simulink model "RefModel_Task"  (R2015b)
settings: configuration reference "CenterOutReachConfigSet" (kept outside this file)
undefined symbols (not defined in the file or in its folder): SimulinkParameter_TunableConditionRepeats, SimulinkParameter_TunableConditions, SimulinkParameter_TunableDataLoggerInfo, SimulinkParameter_TunableNextTrialId, SimulinkParameter_TunableParam, SimulinkParameter_TunableTaskControl
libraries: libBusSerialize x7, libUtilities x1, dspsrcs4 x1
(part 1 of 3)
settings Model: SimulationMode=external  Creator=djoshea  LastModifiedBy=shenoylab
settings ConfigSetRef: SourceLocation=Base Workspace

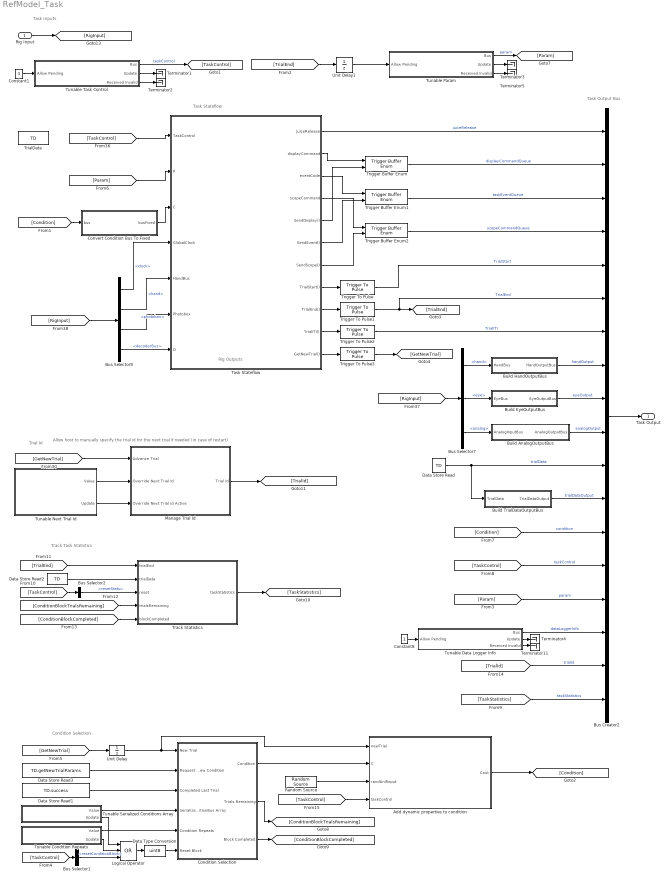
== system RefModel_Task ==
  note: Task Stateflow
  note: Rig Outputs
  note: Task Inputs
  note: Condition Selection
  note: Trial Id
  note: Allow host to manually specify the trial id for the next trial if needed (in case of restart)
  note: Track Task Statistics
  note: Task Output Bus
  Rig Input : Inport  OutDataTypeStr=Bus: RigInputBus  PortDimensions=1  SampleTime=[0.001,0]  Interpolate=off  BusOutputAsStruct=on
  Add dynamic properties to condition : MATLAB Function  TreatAsAtomicUnit=on
  Build AnalogOutputBus : Subsystem
  Build EyeOutputBus : Subsystem
  Build HandOutputBus : Subsystem
  Build TrialDataOutputBus : Subsystem
  Bus Creator2 : BusCreator  Inputs=18
  Bus Selector1 : BusSelector  OutputSignals=resetConditionBlock
  Bus Selector2 : BusSelector  OutputSignals=resetStats
  Bus Selector7 : BusSelector  OutputSignals=hand,eye,analog
  Bus Selector9 : BusSelector  OutputSignals=clock,hand,analog.photobox,decoderBus
  Condition Selection : Subsystem
  Constant1 : Constant  OutDataTypeStr=uint8
  Constant8 : Constant  OutDataTypeStr=uint8
  Convert Condition Bus To Fixed : MATLAB Function  AncestorBlock=libBusSerialize/MATLAB Function1  TreatAsAtomicUnit=on  mask(Drop Variable Length Signals From Bus){busType=Bus: ConditionBus, busFixedType=Bus: ConditionFixedBus}
      mask prompts: busType "Bus Type (Input):"; busFixedType "Bus Type (Output):"
      mask help:
      | This block takes as input a bus with some variable length signals, drops all variable length signals from the bus and outputs a bus with the specified type (second drop-down). This is accomplished by calling the appropriate model packaged code function for this bus.
      |
      | See BusSerialize.createBusBaseWorkspaceWithFixedSizeSignalsOnly and BusSerialize.writeDropVariableLengthSignalsFromBusModelPackagedCode.
      mask init:
      | BusSerialize.maskDropVariableLengthSignalsFromBusBlockUpdate(gcb)
  Data Store Read : DataStoreRead  DataStoreName=TD
  Data Store Read1 : DataStoreRead  DataStoreName=TD  DataStoreElements=TD.success
  Data Store Read2 : DataStoreRead  DataStoreName=TD
  Data Store Read3 : DataStoreRead  DataStoreName=TD  DataStoreElements=TD.getNewTrialParams
  Data Type Conversion : DataTypeConversion  OutDataTypeStr=uint8
  Logical Operator : Logic  Operator=OR  Inputs=3  AllPortsSameDT=off  OutDataTypeStr=boolean
  Manage Trial Id : Subsystem
  Random Source : dspsrcs4/Random Source  SrcType=Uniform  NormMethod=Ziggurat  CltLength=12  MinVal=0  MaxVal=1  MeanVal=0  VarVal=1  RepMode=Not repeatable  rawSeed=1  IsInherit=off  SampMode=Discrete  SampTime=0.001  SampFrame=1  DataType=Double  OutComplex=Real  OutputFrames=on
  Task Stateflow : Stateflow chart  TreatAsAtomicUnit=on
  Terminator{1..5,11} (6 alike) : Terminator
  Track Statistics : MATLAB Function  TreatAsAtomicUnit=on
  TrialData : DataStoreMemory  DataStoreName=TD  ReadBeforeWriteMsg=warning  WriteAfterWriteMsg=warning  WriteAfterReadMsg=warning  OutDataTypeStr=Bus: TrialDataBus
  Trigger Buffer Enum : libBusSerialize/Trigger Buffer Enum  bufferType=Enum: DisplayCommand
  Trigger Buffer Enum1 : libBusSerialize/Trigger Buffer Enum  bufferType=Enum: TaskEvent
  Trigger Buffer Enum2 : libBusSerialize/Trigger Buffer Enum  bufferType=Enum: ScopeCommand
  Trigger To Pulse{,1..3} (4 alike) : libBusSerialize/Trigger To Pulse
  Tunable Condition Repeats : Subsystem  AncestorBlock=libBusSerialize/Tunable Parameter  mask(BusSerialize Tunable Parameter Block){paramName='TunableConditionRepeats'}
      mask prompts: paramName "Parameter Name"
      mask help: This block provides the value of a tunable Simulink.Parameter into the model. Since tunable parameters with xPC target can only be doubles, the functions BusSerialize.createTunableParameter and BusSerialize.setTunableParameter automatically handle typecasting and update counter insertion, and this block handles update detection, typecasting, and reshaping back to the original form. Currently, variable size parameters are not supported.
      mask init:
      | BusSerialize.maskTunableParameterBlockUpdate(gcb);
      mask Display:
      | port_label('output', 1, paramName)
      | port_label('output', 2, 'Update');
  Tunable Data Logger Info : Subsystem  AncestorBlock=libBusSerialize/Serialized Bus Tunable Parameter  mask(BusSerialize Tunable Parameter Block){paramName='TunableDataLoggerInfo'}
      mask prompts: paramName "Parameter Name"
      mask help: This block provides the value of a tunable Simulink.Parameter into the model. Since tunable parameters with xPC target can only be doubles, the functions BusSerialize.createTunableParameter and BusSerialize.setTunableParameter automatically handle typecasting and update counter insertion, and this block handles update detection, typecasting, and reshaping back to the original form. Currently, variable size parameters are not supported.
      mask init:
      | BusSerialize.maskSerializedBusTunableParameterBlockUpdate(gcb);
      mask Display:
      | port_label('output', 1, paramName);
      | port_label('output', 2, 'Update');
      | port_label('output', 3, 'Received Invalid');
      | port_label('input', 1, 'Allow Pending');
  Tunable Next Trial Id : Subsystem  AncestorBlock=libBusSerialize/Tunable Parameter  mask(BusSerialize Tunable Parameter Block){paramName='TunableNextTrialId'}
      mask prompts: paramName "Parameter Name"
      mask help: This block provides the value of a tunable Simulink.Parameter into the model. Since tunable parameters with xPC target can only be doubles, the functions BusSerialize.createTunableParameter and BusSerialize.setTunableParameter automatically handle typecasting and update counter insertion, and this block handles update detection, typecasting, and reshaping back to the original form. Currently, variable size parameters are not supported.
      mask init:
      | BusSerialize.maskTunableParameterBlockUpdate(gcb);
      mask Display:
      | port_label('output', 1, paramName)
      | port_label('output', 2, 'Update');
  Tunable Param : Subsystem  AncestorBlock=libBusSerialize/Serialized Bus Tunable Parameter  mask(BusSerialize Tunable Parameter Block){paramName='TunableParam'}
      mask prompts: paramName "Parameter Name"
      mask help: This block provides the value of a tunable Simulink.Parameter into the model. Since tunable parameters with xPC target can only be doubles, the functions BusSerialize.createTunableParameter and BusSerialize.setTunableParameter automatically handle typecasting and update counter insertion, and this block handles update detection, typecasting, and reshaping back to the original form. Currently, variable size parameters are not supported.
      mask init:
      | BusSerialize.maskSerializedBusTunableParameterBlockUpdate(gcb);
      mask Display:
      | port_label('output', 1, paramName);
      | port_label('output', 2, 'Update');
      | port_label('output', 3, 'Received Invalid');
      | port_label('input', 1, 'Allow Pending');
  Tunable Serialized Conditions Array : Subsystem  AncestorBlock=libBusSerialize/Tunable Serialized Conditions Array  mask(BusSerialize Tunable Parameter Variable Length Bus Array Block){paramName='TunableConditions'}
      mask prompts: paramName "Parameter Name"
      mask help:
      | This block provides the value of a tunable Simulink.Parameter into the model. Since tunable parameters with xPC target can only be doubles, the functions BusSerialize.createTunableParameter and BusSerialize.setTunableParameter automatically handle typecasting and update counter insertion, and this block handles update detection, typecasting, and reshaping back to the original form. Currently, variable size parameters are not supported.
      |
      | This block specifically extracts a serialized variable length bus array, which can then be passed into the variable length bus array element extractor block.
      mask init:
      | BusSerialize.maskTunableParameterVariableLengthBusArrayBlockUpdate(gcb);
      mask Display:
      | port_label('output', 1, paramName)
      | port_label('output', 2, 'Update');
  Tunable Task Control : Subsystem  AncestorBlock=libBusSerialize/Serialized Bus Tunable Parameter  mask(BusSerialize Tunable Parameter Block){paramName='TunableTaskControl'}
      mask prompts: paramName "Parameter Name"
      mask help: This block provides the value of a tunable Simulink.Parameter into the model. Since tunable parameters with xPC target can only be doubles, the functions BusSerialize.createTunableParameter and BusSerialize.setTunableParameter automatically handle typecasting and update counter insertion, and this block handles update detection, typecasting, and reshaping back to the original form. Currently, variable size parameters are not supported.
      mask init:
      | BusSerialize.maskSerializedBusTunableParameterBlockUpdate(gcb);
      mask Display:
      | port_label('output', 1, paramName);
      | port_label('output', 2, 'Update');
      | port_label('output', 3, 'Received Invalid');
      | port_label('input', 1, 'Allow Pending');
  Unit Delay : UnitDelay  SampleTime=-1
  Unit Delay1 : UnitDelay  SampleTime=-1
  Task Output : Outport  OutDataTypeStr=Bus: TaskOutputBus  PortDimensions=1  SampleTime=[0.001,0]  BusOutputAsStruct=on
  wires:
  Task Stateflow/5(SendDisplay()) -> Trigger Buffer Enum/2
  Task Stateflow/9(TrialEnd()) -> Trigger To Pulse1/1
  Rig Input/1 -> [RigInput]
  Task Stateflow/2(displayCommand) -> Trigger Buffer Enum/1
  Trigger Buffer Enum1/1 -> Bus Creator2/3  "taskEventQueue"
  Task Stateflow/8(TrialStart()) -> Trigger To Pulse/1
  Task Stateflow/3(eventCode) -> Trigger Buffer Enum1/1
  Task Stateflow/6(SendEvent()) -> Trigger Buffer Enum1/2
  Trigger Buffer Enum/1 -> Bus Creator2/2  "displayCommandQueue"
  Task Stateflow/10(TrialITI()) -> Trigger To Pulse2/1
  Bus Selector9/1 -> Task Stateflow/4(GlobalClock)  "<clock>"
  [RigInput] -> Bus Selector9/1
  Bus Selector9/2 -> Task Stateflow/5(HandBus)  "<hand>"
  Bus Selector9/3 -> Task Stateflow/6(Photobox)  "<photobox>"
  Trigger To Pulse/1 -> Bus Creator2/5  "TrialStart"
  Trigger To Pulse1/1 -> Bus Creator2/6, [TrialEnd]  "TrialEnd"
  Trigger To Pulse2/1 -> Bus Creator2/7  "TrialITI"
  Task Stateflow/1(JuiceRelease) -> Bus Creator2/1  "juiceRelease"
  [RigInput] -> Bus Selector7/1
  Bus Selector7/1 -> Build HandOutputBus/1(HandBus)  "<hand>"
  Build HandOutputBus/1(HandOutputBus) -> Bus Creator2/8  "handOutput"
  Build EyeOutputBus/1(EyeOutputBus) -> Bus Creator2/9  "eyeOutput"
  Bus Selector7/2 -> Build EyeOutputBus/1(EyeBus)  "<eye>"
  Build AnalogOutputBus/1(AnalogOutputBus) -> Bus Creator2/10  "analogOutput"
  Bus Selector7/3 -> Build AnalogOutputBus/1(AnalogInputBus)  "<analog>"
  Bus Creator2/1 -> Task Output/1
  Trigger To Pulse3/1 -> [GetNewTrial]
  Task Stateflow/11(GetNewTrial()) -> Trigger To Pulse3/1
  [GetNewTrial] -> Manage Trial Id/1(Advance Trial)
  Data Store Read/1 -> Bus Creator2/11, Build TrialDataOutputBus/1(TrialData)  "trialData"
  Build TrialDataOutputBus/1(TrialDataOutput) -> Bus Creator2/12  "trialDataOutput"
  [TaskControl] -> Bus Creator2/14  "taskControl"
  [Param] -> Bus Creator2/15  "param"
  Tunable Data Logger Info/1(Bus) -> Bus Creator2/16  "dataLoggerInfo"
  Condition Selection/1(Condition) -> Add dynamic properties to condition/2(C)
  [Condition] -> Convert Condition Bus To Fixed/1(bus)
  Constant1/1 -> Tunable Task Control/1(Allow Pending)
  Tunable Task Control/3(Received Invalid) -> Terminator2/1
  Tunable Param/3(Received Invalid) -> Terminator5/1
  Tunable Param/1(Bus) -> [Param]  "param"
  Logical Operator/1 -> Data Type Conversion/1
  Tunable Serialized Conditions Array/1(Value) -> Condition Selection/4(Serialized ConditionBus Array)
  Constant8/1 -> Tunable Data Logger Info/1(Allow Pending)
  Tunable Data Logger Info/3(Received Invalid) -> Terminator11/1
  Tunable Condition Repeats/1(Value) -> Condition Selection/5(Condition Repeats)
  [TrialEnd] -> Unit Delay1/1
  Unit Delay1/1 -> Tunable Param/1(Allow Pending)
  Manage Trial Id/1(Trial Id) -> [TrialId]
  [GetNewTrial] -> Unit Delay/1
  Condition Selection/2(Trials Remaining) -> [ConditionBlockTrialsRemaining]
  Unit Delay/1 -> Add dynamic properties to condition/1(newTrial), Condition Selection/1(New Trial)
  Data Store Read1/1 -> Condition Selection/3(Completed Last Trial)
  Tunable Task Control/1(Bus) -> [TaskControl]  "taskControl"
  Tunable Task Control/2(Update) -> Terminator1/1
  Tunable Param/2(Update) -> Terminator3/1
  Data Type Conversion/1 -> Condition Selection/6(Reset Block)
  Tunable Serialized Conditions Array/2(Update) -> Logical Operator/1
  Tunable Condition Repeats/2(Update) -> Logical Operator/2
  Tunable Data Logger Info/2(Update) -> Terminator4/1
  [TaskControl] -> Task Stateflow/1(TaskControl)
  Tunable Next Trial Id/1(Value) -> Manage Trial Id/2(Override Next Trial Id)
  [TaskControl] -> Bus Selector1/1
  Bus Selector1/1 -> Logical Operator/3  "<resetConditionBlock>"
  [Param] -> Task Stateflow/2(P)
  Tunable Next Trial Id/2(Update) -> Manage Trial Id/3(Override Next Trial Id Active)
  [Condition] -> Bus Creator2/13  "condition"
  [TrialEnd] -> Track Statistics/1(trialEnd)
  Data Store Read2/1 -> Track Statistics/2(trialData)
  Condition Selection/3(Block Completed) -> [ConditionBlockCompleted]
  [TaskStatistics] -> Bus Creator2/18  "taskStatistics"
  [TaskControl] -> Bus Selector2/1
  Bus Selector2/1 -> Track Statistics/3(reset)  "<resetStats>"
  [ConditionBlockTrialsRemaining] -> Track Statistics/4(trialsRemaining)
  [ConditionBlockCompleted] -> Track Statistics/5(blockCompleted)
  Track Statistics/1(taskStatistics) -> [TaskStatistics]
  [TrialId] -> Bus Creator2/17  "trialId"
  Convert Condition Bus To Fixed/1(busFixed) -> Task Stateflow/3(C)
  Data Store Read3/1 -> Condition Selection/2(Request New Condition)
  Trigger Buffer Enum2/1 -> Bus Creator2/4  "scopeCommandQueue"
  Task Stateflow/4(scopeCommand) -> Trigger Buffer Enum2/1
  Task Stateflow/7(SendScope()) -> Trigger Buffer Enum2/2
  Random Source/1 -> Add dynamic properties to condition/3(randUnifInput)
  [TaskControl] -> Add dynamic properties to condition/4(taskControl)
  Add dynamic properties to condition/1(Cout) -> [Condition]
  Bus Selector9/4 -> Task Stateflow/7(D)  "<decoderBus>"

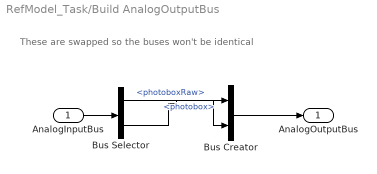
== system RefModel_Task/Build AnalogOutputBus ==
  note: These are swapped so the buses won't be
      | identical
  AnalogInputBus : Inport  OutDataTypeStr=Bus: AnalogInputBus  PortDimensions=1
  Bus Creator : BusCreator  Inputs=2  OutDataTypeStr=Bus: AnalogOutputBus  NonVirtualBus=on
  Bus Selector : BusSelector  OutputSignals=photoboxRaw,photobox
  AnalogOutputBus : Outport  OutDataTypeStr=Bus: AnalogOutputBus  PortDimensions=1
  wires:
  Bus Creator/1 -> AnalogOutputBus/1
  Bus Selector/1 -> Bus Creator/2  "<photoboxRaw>"
  Bus Selector/2 -> Bus Creator/1  "<photobox>"
  AnalogInputBus/1 -> Bus Selector/1

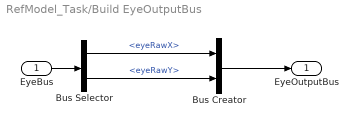
== system RefModel_Task/Build EyeOutputBus ==
  EyeBus : Inport  OutDataTypeStr=Bus: EyeInputBus
  Bus Creator : BusCreator  Inputs=2  OutDataTypeStr=Bus: EyeOutputBus  NonVirtualBus=on
  Bus Selector : BusSelector  OutputSignals=eyeRawX,eyeRawY
  EyeOutputBus : Outport  OutDataTypeStr=Bus: EyeOutputBus
  wires:
  Bus Creator/1 -> EyeOutputBus/1
  Bus Selector/1 -> Bus Creator/1  "<eyeRawX>"
  Bus Selector/2 -> Bus Creator/2  "<eyeRawY>"
  EyeBus/1 -> Bus Selector/1

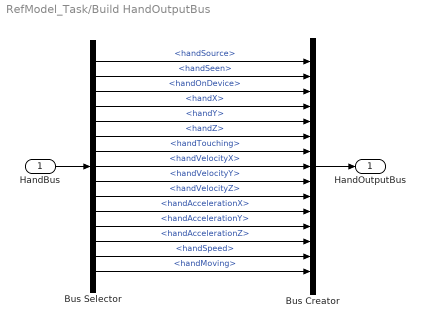
== system RefModel_Task/Build HandOutputBus ==
  HandBus : Inport  OutDataTypeStr=Bus: HandBus
  Bus Creator : BusCreator  Inputs=15  OutDataTypeStr=Bus: HandOutputBus  NonVirtualBus=on
  Bus Selector : BusSelector  OutputSignals=handSource,handSeen,handOnDevice,handX,handY,handZ,handTouching,handVelocityX,handVelocityY,handVelocityZ,handAccelerationX,handAccelerationY,handAccelerationZ,handSpeed,handMoving
  HandOutputBus : Outport  OutDataTypeStr=Bus: HandOutputBus
  wires:
  Bus Creator/1 -> HandOutputBus/1
  Bus Selector/10 -> Bus Creator/10  "<handVelocityZ>"
  Bus Selector/6 -> Bus Creator/6  "<handZ>"
  Bus Selector/7 -> Bus Creator/7  "<handTouching>"
  Bus Selector/8 -> Bus Creator/8  "<handVelocityX>"
  Bus Selector/3 -> Bus Creator/3  "<handOnDevice>"
  Bus Selector/4 -> Bus Creator/4  "<handX>"
  Bus Selector/9 -> Bus Creator/9  "<handVelocityY>"
  Bus Selector/5 -> Bus Creator/5  "<handY>"
  Bus Selector/1 -> Bus Creator/1  "<handSource>"
  Bus Selector/2 -> Bus Creator/2  "<handSeen>"
  HandBus/1 -> Bus Selector/1
  Bus Selector/11 -> Bus Creator/11  "<handAccelerationX>"
  Bus Selector/12 -> Bus Creator/12  "<handAccelerationY>"
  Bus Selector/13 -> Bus Creator/13  "<handAccelerationZ>"
  Bus Selector/14 -> Bus Creator/14  "<handSpeed>"
  Bus Selector/15 -> Bus Creator/15  "<handMoving>"

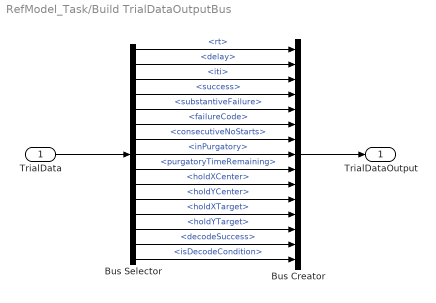
== system RefModel_Task/Build TrialDataOutputBus ==
  TrialData : Inport  OutDataTypeStr=Bus: TrialDataBus
  Bus Creator : BusCreator  Inputs=15  OutDataTypeStr=Bus: TrialDataOutputBus  NonVirtualBus=on
  Bus Selector : BusSelector  OutputSignals=rt,delay,iti,success,substantiveFailure,failureCode,consecutiveNoStarts,inPurgatory,purgatoryTimeRemaining,holdXCenter,holdYCenter,holdXTarget,holdYTarget,decodeSuccess,isDecodeCondition
  TrialDataOutput : Outport  OutDataTypeStr=Bus: TrialDataOutputBus
  wires:
  Bus Creator/1 -> TrialDataOutput/1
  TrialData/1 -> Bus Selector/1
  Bus Selector/1 -> Bus Creator/1  "<rt>"
  Bus Selector/2 -> Bus Creator/2  "<delay>"
  Bus Selector/3 -> Bus Creator/3  "<iti>"
  Bus Selector/4 -> Bus Creator/4  "<success>"
  Bus Selector/5 -> Bus Creator/5  "<substantiveFailure>"
  Bus Selector/6 -> Bus Creator/6  "<failureCode>"
  Bus Selector/8 -> Bus Creator/8  "<inPurgatory>"
  Bus Selector/7 -> Bus Creator/7  "<consecutiveNoStarts>"
  Bus Selector/9 -> Bus Creator/9  "<purgatoryTimeRemaining>"
  Bus Selector/10 -> Bus Creator/10  "<holdXCenter>"
  Bus Selector/11 -> Bus Creator/11  "<holdYCenter>"
  Bus Selector/12 -> Bus Creator/12  "<holdXTarget>"
  Bus Selector/13 -> Bus Creator/13  "<holdYTarget>"
  Bus Selector/14 -> Bus Creator/14  "<decodeSuccess>"
  Bus Selector/15 -> Bus Creator/15  "<isDecodeCondition>"

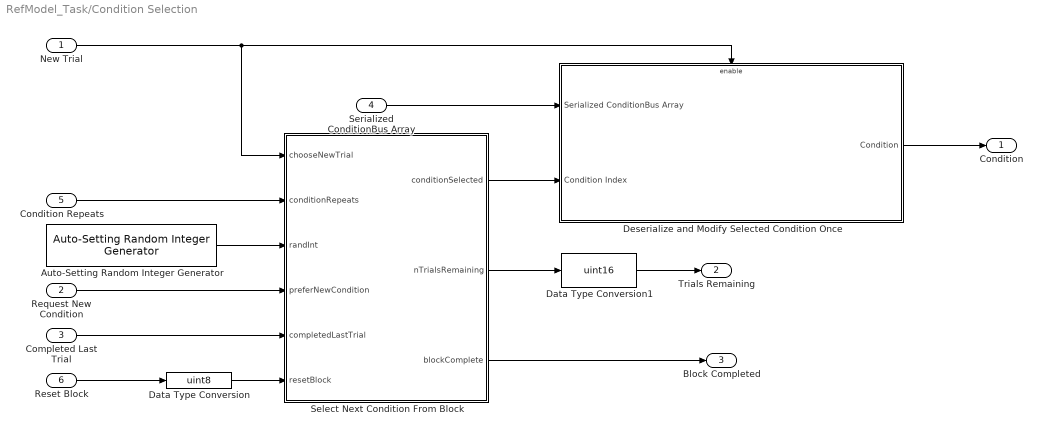
== system RefModel_Task/Condition Selection ==
  New Trial : Inport  OutDataTypeStr=uint8  PortDimensions=1
  Request New Condition : Inport  Port=2  OutDataTypeStr=uint8  PortDimensions=1
  Completed Last Trial : Inport  Port=3  OutDataTypeStr=uint8  PortDimensions=1
  Serialized ConditionBus Array : Inport  Port=4  OutDataTypeStr=uint8
  Condition Repeats : Inport  Port=5  OutDataTypeStr=uint16
  Reset Block : Inport  Port=6  OutDataTypeStr=uint8  PortDimensions=1
  Auto-Setting Random Integer Generator : libUtilities/Auto-Setting Random Integer Generator  mul=2^32  Ts=0.001  outDataType=uint32
  Data Type Conversion : DataTypeConversion  OutDataTypeStr=uint8
  Data Type Conversion1 : DataTypeConversion  OutDataTypeStr=uint16
  Deserialize and Modify Selected Condition Once : Subsystem
  Select Next Condition From Block : MATLAB Function  TreatAsAtomicUnit=on
  Condition : Outport  OutDataTypeStr=Bus: ConditionBus
  Trials Remaining : Outport  Port=2  OutDataTypeStr=uint16  InitialOutput=0
  Block Completed : Outport  Port=3  OutDataTypeStr=uint8  PortDimensions=1  InitialOutput=0
  wires:
  Select Next Condition From Block/3(blockComplete) -> Block Completed/1
  Reset Block/1 -> Data Type Conversion/1
  Auto-Setting Random Integer Generator/1 -> Select Next Condition From Block/3(randInt)
  Condition Repeats/1 -> Select Next Condition From Block/2(conditionRepeats)
  Data Type Conversion/1 -> Select Next Condition From Block/6(resetBlock)
  Select Next Condition From Block/2(nTrialsRemaining) -> Data Type Conversion1/1
  Data Type Conversion1/1 -> Trials Remaining/1
  Completed Last Trial/1 -> Select Next Condition From Block/5(completedLastTrial)
  Select Next Condition From Block/1(conditionSelected) -> Deserialize and Modify Selected Condition Once/2(Condition Index)
  Deserialize and Modify Selected Condition Once/1(Condition) -> Condition/1
  New Trial/1 -> Select Next Condition From Block/1(chooseNewTrial), Deserialize and Modify Selected Condition Once/Enable
  Serialized ConditionBus Array/1 -> Deserialize and Modify Selected Condition Once/1(Serialized ConditionBus Array)
  Request New Condition/1 -> Select Next Condition From Block/4(preferNewCondition)

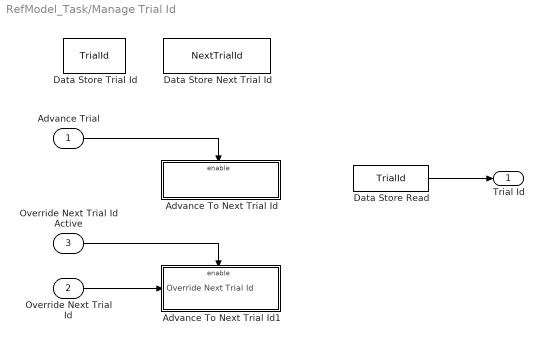
== system RefModel_Task/Manage Trial Id ==
  Advance Trial : Inport  OutDataTypeStr=uint8
  Override Next Trial Id : Inport  Port=2  OutDataTypeStr=uint32
  Override Next Trial Id Active : Inport  Port=3  OutDataTypeStr=uint8
  Advance To Next Trial Id : Subsystem
  Advance To Next Trial Id1 : Subsystem
  Data Store Next Trial Id : DataStoreMemory  DataStoreName=NextTrialId  ReadBeforeWriteMsg=warning  WriteAfterWriteMsg=warning  WriteAfterReadMsg=warning  OutDataTypeStr=uint32  Dimensions=1
  Data Store Read : DataStoreRead  DataStoreName=TrialId
  Data Store Trial Id : DataStoreMemory  DataStoreName=TrialId  ReadBeforeWriteMsg=warning  WriteAfterWriteMsg=warning  WriteAfterReadMsg=warning  OutDataTypeStr=uint32  Dimensions=1
  Trial Id : Outport
  wires:
  Advance Trial/1 -> Advance To Next Trial Id/Enable
  Override Next Trial Id Active/1 -> Advance To Next Trial Id1/Enable
  Override Next Trial Id/1 -> Advance To Next Trial Id1/1(Override Next Trial Id)
  Data Store Read/1 -> Trial Id/1

== system RefModel_Task/Tunable Condition Repeats ==
  Deserialize Parameter : MATLAB Function  TreatAsAtomicUnit=on
  Parameter Value : Constant  Value=SimulinkParameter_TunableConditionRepeats  OutDataTypeStr=double
  Value : Outport
  Update : Outport  Port=2
  wires:
  Parameter Value/1 -> Deserialize Parameter/1(valAsDouble)
  Deserialize Parameter/2(update) -> Update/1
  Deserialize Parameter/1(value) -> Value/1

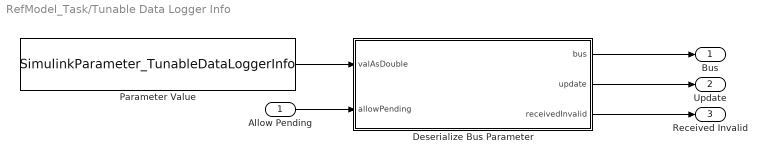
== system RefModel_Task/Tunable Data Logger Info ==
  Allow Pending : Inport
  Deserialize Bus Parameter : MATLAB Function  TreatAsAtomicUnit=on
  Parameter Value : Constant  Value=SimulinkParameter_TunableDataLoggerInfo  OutDataTypeStr=double
  Bus : Outport  PortDimensions=1
  Update : Outport  Port=2  OutDataTypeStr=uint8  PortDimensions=1
  Received Invalid : Outport  Port=3  OutDataTypeStr=uint8  PortDimensions=1
  wires:
  Parameter Value/1 -> Deserialize Bus Parameter/1(valAsDouble)
  Allow Pending/1 -> Deserialize Bus Parameter/2(allowPending)
  Deserialize Bus Parameter/3(receivedInvalid) -> Received Invalid/1
  Deserialize Bus Parameter/1(bus) -> Bus/1
  Deserialize Bus Parameter/2(update) -> Update/1

== system RefModel_Task/Tunable Next Trial Id ==
  Deserialize Parameter : MATLAB Function  TreatAsAtomicUnit=on
  Parameter Value : Constant  Value=SimulinkParameter_TunableNextTrialId  OutDataTypeStr=double
  Value : Outport
  Update : Outport  Port=2
  wires:
  Parameter Value/1 -> Deserialize Parameter/1(valAsDouble)
  Deserialize Parameter/2(update) -> Update/1
  Deserialize Parameter/1(value) -> Value/1

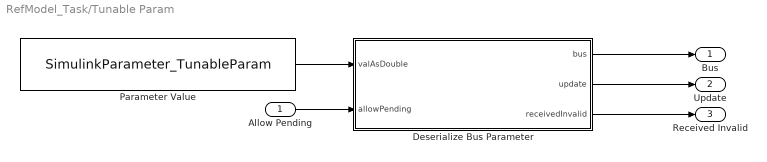
== system RefModel_Task/Tunable Param ==
  Allow Pending : Inport
  Deserialize Bus Parameter : MATLAB Function  TreatAsAtomicUnit=on
  Parameter Value : Constant  Value=SimulinkParameter_TunableParam  OutDataTypeStr=double
  Bus : Outport  PortDimensions=1
  Update : Outport  Port=2  OutDataTypeStr=uint8  PortDimensions=1
  Received Invalid : Outport  Port=3  OutDataTypeStr=uint8  PortDimensions=1
  wires:
  Parameter Value/1 -> Deserialize Bus Parameter/1(valAsDouble)
  Allow Pending/1 -> Deserialize Bus Parameter/2(allowPending)
  Deserialize Bus Parameter/3(receivedInvalid) -> Received Invalid/1
  Deserialize Bus Parameter/1(bus) -> Bus/1
  Deserialize Bus Parameter/2(update) -> Update/1

== system RefModel_Task/Tunable Serialized Conditions Array ==
  Deserialize Parameter : MATLAB Function  TreatAsAtomicUnit=on
  Parameter Value : Constant  Value=SimulinkParameter_TunableConditions  OutDataTypeStr=double
  Value : Outport
  Update : Outport  Port=2
  wires:
  Deserialize Parameter/1(value) -> Value/1
  Deserialize Parameter/2(update) -> Update/1
  Parameter Value/1 -> Deserialize Parameter/1(valAsDouble)

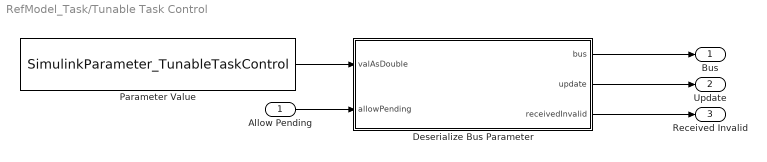
== system RefModel_Task/Tunable Task Control ==
  Allow Pending : Inport
  Deserialize Bus Parameter : MATLAB Function  TreatAsAtomicUnit=on
  Parameter Value : Constant  Value=SimulinkParameter_TunableTaskControl  OutDataTypeStr=double
  Bus : Outport  PortDimensions=1
  Update : Outport  Port=2  OutDataTypeStr=uint8  PortDimensions=1
  Received Invalid : Outport  Port=3  OutDataTypeStr=uint8  PortDimensions=1
  wires:
  Parameter Value/1 -> Deserialize Bus Parameter/1(valAsDouble)
  Allow Pending/1 -> Deserialize Bus Parameter/2(allowPending)
  Deserialize Bus Parameter/3(receivedInvalid) -> Received Invalid/1
  Deserialize Bus Parameter/1(bus) -> Bus/1
  Deserialize Bus Parameter/2(update) -> Update/1

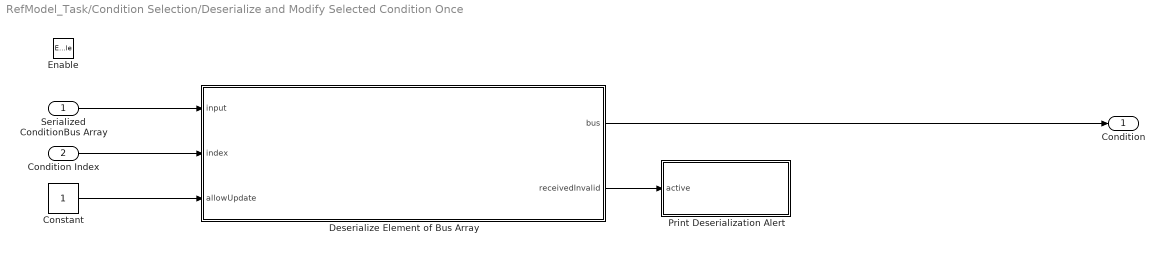
== system RefModel_Task/Condition Selection/Deserialize and Modify Selected Condition Once ==
  Serialized ConditionBus Array : Inport
  Condition Index : Inport  Port=2
  Enable : EnablePort  PropagateVarSize=During execution
  Constant : Constant  OutDataTypeStr=uint8
  Deserialize Element of Bus Array : MATLAB Function  AncestorBlock=libBusSerialize/Deserialize Element of Bus Array  TreatAsAtomicUnit=on  mask(BusSerialize: deserialize a single element of a serialized bus array){busType=Bus: ConditionBus, inputVariable=off}
      mask prompts: busType "Bus Type:"; inputVariable "Input Variable Length"
      mask help:
      | Given a bus array serialized with BusSerialize.serializeVariableLengthBusArray, this block deserializes a specific element of that bus array. This allows bus arrays to be deserialized even when the bus contains variable length elements (or the array is of variable length), which implies that Simulink cannot currently handle the bus array.
      |
      | Select the bus type below to deserialize into.
      mask init:
      | BusSerialize.maskDeserializeVariableLengthBusArrayBlockUpdate(gcb)
  Print Deserialization Alert : MATLAB Function  TreatAsAtomicUnit=on
  Condition : Outport  SourceOfInitialOutputValue=Input signal
  wires:
  Serialized ConditionBus Array/1 -> Deserialize Element of Bus Array/1(input)
  Deserialize Element of Bus Array/1(bus) -> Condition/1
  Condition Index/1 -> Deserialize Element of Bus Array/2(index)
  Deserialize Element of Bus Array/2(receivedInvalid) -> Print Deserialization Alert/1(active)
  Constant/1 -> Deserialize Element of Bus Array/3(allowUpdate)

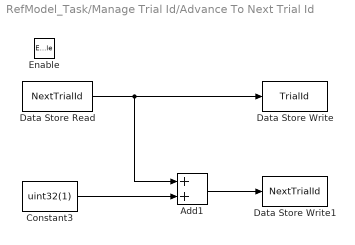
== system RefModel_Task/Manage Trial Id/Advance To Next Trial Id ==
  Enable : EnablePort
  Add1 : Sum
  Constant3 : Constant  Value=uint32(1)
  Data Store Read : DataStoreRead  DataStoreName=NextTrialId
  Data Store Write : DataStoreWrite  DataStoreName=TrialId
  Data Store Write1 : DataStoreWrite  DataStoreName=NextTrialId
  wires:
  Add1/1 -> Data Store Write1/1
  Constant3/1 -> Add1/2
  Data Store Read/1 -> Add1/1, Data Store Write/1

== system RefModel_Task/Manage Trial Id/Advance To Next Trial Id1 ==
  Override Next Trial Id : Inport
  Enable : EnablePort
  Data Store Write1 : DataStoreWrite  DataStoreName=NextTrialId
  wires:
  Override Next Trial Id/1 -> Data Store Write1/1

== matlab function RefModel_Task/Tunable Param/Deserialize Bus Parameter ==
  data: valAsDouble input double; bus output Bus: ParamBus size=1; update output uint8 size=1; allowPending input uint8 size=1; receivedInvalid output uint8 size=1
function [bus, update, receivedInvalid] = deserializeBusParameter(valAsDouble, allowPending)
%#codegen

    % typecast to bytes
    valAsBytes = typecast(valAsDouble, 'uint8');

    % use the first byte as updateCounter, check for whether counter has been incremented
    thisCounter = valAsBytes(1);
    persistent pLastCounter;
    if isempty(pLastCounter)
        pLastCounter = thisCounter;
    end
    if pLastCounter ~= thisCounter
        recvUpdate = uint8(1);
        pLastCounter = thisCounter;
    else
        recvUpdate = uint8(0);
    end
    startOffset = 2;

    % external cached output for when allowPending 
    persistent pBusOut;
    if isempty(pBusOut)
        pBusOut = initializeBus_ParamBus();
    end

    % parse incoming bytes if allowing updates
    receivedInvalid = uint8(0);
    if allowPending
        [bus, valid] = deserializeBus_ParamBus(valAsBytes, startOffset);
        if valid
            % update internal cache
            pBusOut = bus;
        else
            % don't update internal cache, output internal cache
            bus = pBusOut;
            receivedInvalid = uint8(1);
            recvUpdate = uint8(0);
        end
    else
        bus = pBusOut;
    end

    % track whether we have a pending update
    persistent pPending;
    if isempty(pPending), pPending = uint8(0); end
    if recvUpdate
        if allowPending
            % update goes out immediately
            update = uint8(1);
            pPending = uint8(0);
        else
            % queue pending update
            update = uint8(0);
            pPending = uint8(1);
        end
    else
        if allowPending
            % release pending
            update = pPending;
            pPending = uint8(0);
        else
            % do nothing
            update = uint8(0);
        end
    end

    % reset fields marked with .resetImmediately immediately after update
    if ~update
        bus.resetImageDecoder = uint8(0);

    end
end

== matlab function RefModel_Task/Tunable Next Trial Id/Deserialize Parameter ==
  data: valAsDouble input double; value output uint32 size=[1 1]; update output uint8 size=1
function [value, update] = deserializeParameter(valAsDouble)
%#codegen

valAsBytes = typecast(valAsDouble, 'uint8');

% check for whether counter has been incremented
thisCounter = valAsBytes(1);
persistent pLastCounter;
if isempty(pLastCounter)
    pLastCounter = thisCounter;
end
if pLastCounter ~= thisCounter
    update = uint8(1);
    pLastCounter = thisCounter;
else
    update = uint8(0);
end

% typecast and reshape the value
value = reshape(typecast(valAsBytes(double(2):double(5)), 'uint32'), [1 1]);
